simulink model "modelComposerHW"  (R2021a)
settings: Solver=VariableStepAuto  StartTime=0.0  StopTime=300  RelTol=1e-3
undefined symbols (not defined in the file or in its folder): A, N
libraries: hdlBasic x24, xbsIndex_r4 x1, JTAGRuntimeCosim_r4 x1
settings Model: Creator=kv25  LastModifiedBy=kv25

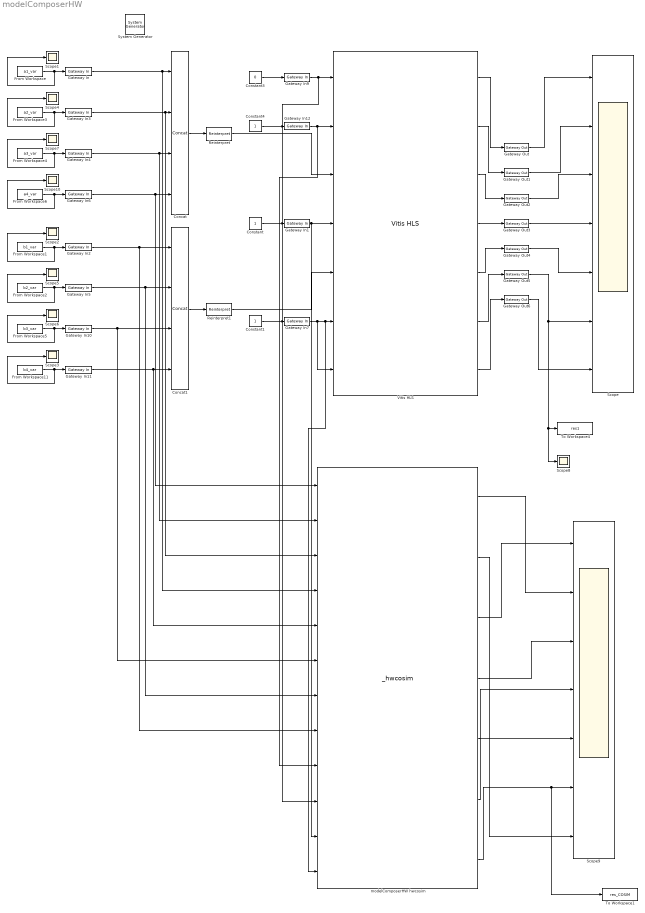
== system modelComposerHW ==
  " System Generator" : xbsIndex_r4/ System Generator  Tag=genX  xilinxfamily=zynq  part=xc7z020  speed=-1  package=clg484  synthesis_tool=Vivado  clock_wrapper=Clock Enables  directory=./netlist2  proj_type=Vivado  Synth_file=Vivado Synthesis Defaults  Impl_file=Vivado Implementation Defaults  testbench=off  simulink_period=1  sysclk_period=10  dcm_input_clock_period=10  incr_netlist=off  trim_vbits=Everywhere in SubSystem  dbl_ovrd=According to Block Masks  core_generation=According to Block Masks  run_coregen=off  deprecated_control=off  eval_field=0  block_type=sysgen
  Concat : hdlBasic/Concat  num_inputs=4  XmcBlockStatus=1  maskContainerNames=group1  block_type=concat  block_config=sysgen:Concat_config
  Concat1 : hdlBasic/Concat  num_inputs=4  XmcBlockStatus=1  maskContainerNames=group1  block_type=concat  block_config=sysgen:Concat_config
  Constant : Constant
  Constant1 : Constant
  Constant3 : Constant  Value=0
  Constant4 : Constant
  From Workspace : FromWorkspace  VariableName=a1_var
  From Workspace1 : FromWorkspace  VariableName=b1_var
  From Workspace11 : FromWorkspace  VariableName=b4_var
  From Workspace2 : FromWorkspace  VariableName=b2_var
  From Workspace3 : FromWorkspace  VariableName=a2_var
  From Workspace4 : FromWorkspace  VariableName=a3_var
  From Workspace5 : FromWorkspace  VariableName=b3_var
  From Workspace6 : FromWorkspace  VariableName=a4_var
  Gateway In{,2..6,10..11} (8 alike) : hdlBasic/Gateway In  gui_display_data_type=Fixed-point  arith_type=Unsigned  n_bits=16  bin_pt=0  preci_type=Single  exp_width=8  frac_width=24  rows=1  columns=1  quantization="Round  (unbiased: +/- Inf)"  overflow=Saturate  period=1  UseAsADC=off  ADCChannel='1'  interface=None  automatic_assignment=on  address_offset=hex2dec('00')  intf_name=''  intf_description=''  default_value=0  timing_constraint=None  locs_specified=off  LOCs={}  io_standard={}  inherit_from_input=off  hdl_port=on  XmcBlockStatus=1  maskContainerNames=group4  block_type=gatewayin  block_config=sysgen:gateway_in_config  block_width_w=590  block_height_w=620  block_width=640  block_height=850
  Gateway In{1,7,9,12} (4 alike) : hdlBasic/Gateway In  gui_display_data_type=Boolean  arith_type=Boolean  n_bits=16  bin_pt=0  preci_type=Single  exp_width=8  frac_width=24  rows=1  columns=1  quantization="Round  (unbiased: +/- Inf)"  overflow=Saturate  period=1  UseAsADC=off  ADCChannel='1'  interface=None  automatic_assignment=on  address_offset=hex2dec('00')  intf_name=''  intf_description=''  default_value=0  timing_constraint=None  locs_specified=off  LOCs={}  io_standard={}  inherit_from_input=off  hdl_port=on  XmcBlockStatus=1  maskContainerNames=group4  block_type=gatewayin  block_config=sysgen:gateway_in_config  block_width_w=590  block_height_w=620  block_width=640  block_height=850
  Gateway Out{,1..6} (7 alike) : hdlBasic/Gateway Out  inherit_from_input=off  hdl_port=on  rows=1  columns=1  UseAsDAC=off  DACChannel='1'  interface=None  automatic_assignment=on  address_offset=hex2dec('00')  intf_name=''  intf_description=''  timing_constraint=None  locs_specified=off  LOCs={}  io_standard={}  XmcBlockStatus=1  maskContainerNames=group4  block_type=gatewayout  block_config=sysgen:gateway_out_config  block_width_w=590  block_height_w=620  block_width=620  block_height=750
  Reinterpret : hdlBasic/Reinterpret  force_arith_type=on  arith_type=Unsigned  force_bin_pt=off  bin_pt=0  XmcBlockStatus=1  maskContainerNames=group1  block_type=reinterpret  block_config=sysgen:Reinterpret_config
  Reinterpret1 : hdlBasic/Reinterpret  force_arith_type=on  arith_type=Unsigned  force_bin_pt=off  bin_pt=0  XmcBlockStatus=1  maskContainerNames=group1  block_type=reinterpret  block_config=sysgen:Reinterpret_config
  Scope : Scope  NumInputPorts=7
  Scope{1..8,10} (9 alike) : Scope
  Scope9 : Scope  NumInputPorts=7
  To Workspace1 : ToWorkspace  VariableName=res_COSIM  SaveFormat=Timeseries  SampleTime=-1
  To Workspace4 : ToWorkspace  VariableName=res1  SaveFormat=Timeseries  SampleTime=-1
  Vitis HLS : hdlBasic/Vitis HLS  anytable='.\Vitis_HLS\matrixmul\solution1'  fast_sim=on  display_datatype=off  rate_propagation_method=Simulink system period  model_file_path=''  latency=1  block_type=vitis_hls
      settings: infoedit=This block allows including C,C++ and SystemC source files in System Generator for DSP designs.
  modelComposerHW hwcosim : JTAGRuntimeCosim_r4/_hwcosim  clkSrc=Single Stepped  hasCombinationalPath=on  bitfileName=C:\ELEC522\venaik\Project3\project3\netlist2\modelcomposerhw.bit  skipConfig=off  dispPartInfo=off  useZynqReconfigScript=on  cable=Auto Detect  speed=N/A  cablePort=N/A  cableLocation=Local  shareCable=off  xmp=[]  software_settings=[]  design_xtable=|  binDir=[]  engineDll=JTAGCosimEngine.dll  cableWaitTime=10  bscanPos=-1  IRLengths=[]  useWaitBox=1  hasBufgmux=on  Scheme=Cosim  useCmdProc=1  hasProc=0  useImpact=0  printLogFile=0  userChain=2  XmcBlockStatus=0  maskContainerNames=tabcontainer1  block_type=jtagcosim  block_config=Sysgen:hwcosim_block_config
      | {
      |     'clkWrapper' => 'modelcomposerhw',
      |     'burstMode' => false,
      |     'burstFifoDepth' => '1024',
      |     'shared_memories' => {},
      |     'clocksGcd' => 1,
      |     'device' => {
      |       'family' => 'zynq',
      |       'part' => 'xc7z020',
      |       'package' => 'clg484',
      |       'speed' => '-1',
      |     },
      |     'ports' => {
      |       'gateway_in6' => {
      |         'direction' => 'in',
      |         'width' => 16,
      |         'name' => 'gateway_in6',
      |         'period' => 1,
      |         'icon_text' => 'Gateway In6',
      |         'type' => 'UFix_16_0',
      |         'arithmetic_type' => 'xlUnsigned',
      |         'dat_file' => 'modelcomposerhw_gateway_in6.dat',
      |         'bin_pt' => 0,
      |         'addr_offset' => 0,
      |         'bd_port_index' => 0,
      |       },
      |       'gateway_in4' => {
      |         'direction' => 'in',
      |         'width' => 16,
      |         'name' => 'gateway_in4',
      |         'period' => 1,
      |         'icon_text' => 'Gateway In4',
      |         'type' => 'UFix_16_0',
      |         'arithmetic_type' => 'xlUnsigned',
      |         'dat_file' => 'modelcomposerhw_gateway_in4.dat',
      |         'bin_pt' => 0,
      |         'addr_offset' => 4,
      |         'bd_port_index' => 1,
      |       },
      |       'gateway_in3' => {
      |         'direction' => 'in',
      |         'width' => 16,
      |         'name' => 'gateway_in3',
      |         'period' => 1,
      |         'icon_text' => 'Gateway In3',
      |         'type' => 'UFix_16_0',
      |         'arithmetic_type' => 'xlUnsigned',
      |         'dat_file' => 'modelcomposerhw_gateway_in3.dat',
      |         'bin_pt' => 0,
      |         'addr_offset' => 8,
      |         'bd_port_index' => 2,
      |       },
      |       'gateway_in' => {
      |         'direction' => 'in',
      |         'width' => 16,
      |         'name' => 'gateway_in',
      |         'period' => 1,
      |         'icon_text' => 'Gateway In',
      |         'type' => 'UFix_16_0',
      |         'arithmetic_type' => 'xlUnsigned',
      |         'dat_file' => 'modelcomposerhw_gateway_in.dat',
      |         'bin_pt' => 0,
      |         'addr_offset' => 12,
      |         'bd_port_index' => 3,
      |       },
      |       'gateway_in11' => {
      |         'direction' => 'in',
      |         'width' => 16,
      |         'name' => 'gateway_in11',
      |         'period' => 1,
      |         'icon_text' => 'Gateway In11',
      |         'type' => 'UFix_16_0',
      |         'arithmetic_type' => 'xlUnsigned',
      |         'dat_file' => 'modelcomposerhw_gateway_in11.dat',
      |         'bin_pt' => 0,
      |         'addr_offset' => 16,
      |         'bd_port_index' => 4,
      |       },
      |       'gateway_in10' => {
      |         'direction' => 'in',
      |         'width' => 16,
      |         'name' => 'gateway_in10',
      |         'period' => 1,
      |         'icon_text' => 'Gateway In10',
      |         'type' => 'UFix_16_0',
      |         'arithmetic_type' => 'xlUnsigned',
      |         'dat_file' => 'modelcomposerhw_gateway_in10.dat',
      |         'bin_pt' => 0,
      |         'addr_offset' => 20,
      |         'bd_port_index' => 5,
      |       },
      |       'gateway_in5' => {
      |         'direction' => 'in',
      |         'width' => 16,
      |         'name' => 'gateway_in5',
      |         'period' => 1,
      |         'icon_text' => 'Gateway In5',
      |         'type' => 'UFix_16_0',
      |         'arithmetic_type' => 'xlUnsigned',
      |         'dat_file' => 'modelcomposerhw_gateway_in5.dat',
      |         'bin_pt' => 0,
      |         'addr_offset' => 24,
      |         'bd_port_index' => 6,
      |       },
      |       'gateway_in2' => {
      |         'direction' => 'in',
      |         'width' => 16,
      |         'name' => 'gateway_in2',
      |         'period' => 1,
      |         'icon_text' => 'Gateway In2',
      |         'type' => 'UFix_16_0',
      |         'arithmetic_type' => 'xlUnsigned',
      |         'dat_file' => 'modelcomposerhw_gateway_in2.dat',
      |         'bin_pt' => 0,
      |         'addr_offset' => 28,
      |         'bd_port_index' => 7,
      |       },
      |       'gateway_in12' => {
      |         'direction' => 'in',
      |         'width' => 1,
      |         'name' => 'gateway_in12',
      |         'period' => 1,
      |         'icon_text' => 'Gateway In12',
      |         'type' => 'Bool',
      |         'arithmetic_type' => 'xlUnsigned',
      |         'dat_file' => 'modelcomposerhw_gateway_in12.dat',
      |         'bin_pt' => 0,
      |         'addr_offset' => 32,
      |         'bd_port_index' => 8,
      |       },
      |       'gateway_in9' => {
      |         'direction' => 'in',
      |         'width' => 1,
      |         'name' => 'gateway_in9',
      |         'period' => 1,
      |         'icon_text' => 'Gateway In9',
      |         'type' => 'Bool',
      |         'arithmetic_type' => 'xlUnsigned',
      |         'dat_file' => 'modelcomposerhw_gateway_in9.dat',
      |         'bin_pt' => 0,
      |         'addr_offset' => 36,
      |         'bd_port_index' => 9,
      |       },
      |       'gateway_in1' => {
      |         'direction' => 'in',
      |         'width' => 1,
      |         'name' => 'gateway_in1',
      |         'period' => 1,
      |         'icon_text' => 'Gateway In1',
      |         'type' => 'Bool',
      |         'arithmetic_type' => 'xlUnsigned',
      |         'dat_file' => 'modelcomposerhw_gateway_in1.dat',
      |         'bin_pt' => 0,
      |         'addr_offset' => 40,
      |         'bd_port_index' => 10,
      |       },
      |       'gateway_in7' => {
      |         'direction' => 'in',
      |         'width' => 1,
      |         'name' => 'gateway_in7',
      |         'period' => 1,
      |         'icon_text' => 'Gateway In7',
      |         'type' => 'Bool',
      |         'arithmetic_type' => 'xlUnsigned',
      |         'dat_file' => 'modelcomposerhw_gateway_in7.dat',
      |         'bin_pt' => 0,
      |         'addr_offset' => 44,
      |         'bd_port_index' => 11,
      |       },
      |       'gateway_out1' => {
      |         'direction' => 'out',
      |         'width' => 1,
      |         'name' => 'gateway_out1',
      |         'period' => 1,
      |         'icon_text' => 'Gateway Out1',
      |         'type' => 'Bool',
      |         'arithmetic_type' => 'xlUnsigned',
      |         'dat_file' => 'modelcomposerhw_gateway_out1.dat',
      |         'bin_pt' => 0,
      |         'addr_offset' => 48,
      |         'bd_port_index' => 0,
      |       },
      |       'gateway_out6' => {
      |         'direction' => 'out',
      |         'width' => 1,
      |         'name' => 'gateway_out6',
      |         'period' => 1,
      |         'icon_text' => 'Gateway Out6',
      |         'type' => 'Bool',
      |         'arithmetic_type' => 'xlUnsigned',
      |         'dat_file' => 'modelcomposerhw_gateway_out6.dat',
      |         'bin_pt' => 0,
      |         'addr_offset' => 52,
      |         'bd_port_index' => 1,
      |       },
      |       'gateway_out' => {
      |         'direction' => 'out',
      |         'width' => 1,
      |         'name' => 'gateway_out',
      |         'period' => 1,
      |         'icon_text' => 'Gateway Out',
      |         'type' => 'Bool',
      |         'arithmetic_type' => 'xlUnsigned',
      |         'dat_file' => 'modelcomposerhw_gateway_out.dat',
      |         'bin_pt' => 0,
      |         'addr_offset' => 56,
      |         'bd_port_index' => 2,
      |       },
      |       'gateway_out2' => {
      |         'direction' => 'out',
      |         'width' => 1,
      |         'name' => 'gateway_out2',
      |         'period' => 1,
      |         'icon_text' => 'Gateway Out2',
      |         'type' => 'Bool',
      |         'arithmetic_type' => 'xlUnsigned',
      |         'dat_file' => 'modelcomposerhw_gateway_out2.dat',
      |         'bin_pt' => 0,
      |         'addr_offset' => 60,
      |         'bd_port_index' => 3,
      |       },
      |       'gateway_out3' => {
      |         'direction' => 'out',
      |         'width' => 1,
      |         'name' => 'gateway_out3',
      |         'period' => 1,
      |         'icon_text' => 'Gateway Out3',
      |         'type' => 'Bool',
      |         'arithmetic_type' => 'xlUnsigned',
      |         'dat_file' => 'modelcomposerhw_gateway_out3.dat',
      |         'bin_pt' => 0,
      |         'addr_offset' => 64,
      |         'bd_port_index' => 4,
      |       },
      |       'gateway_out4' => {
      |         'direction' => 'out',
      |         'width' => 1,
      |         'name' => 'gateway_out4',
      |         'period' => 1,
      |         'icon_text' => 'Gateway Out4',
      |         'type' => 'Bool',
      |         'arithmetic_type' => 'xlUnsigned',
      |         'dat_file' => 'modelcomposerhw_gateway_out4.dat',
      |         'bin_pt' => 0,
      |         'addr_offset' => 68,
      |         'bd_port_index' => 5,
      |       },
      |       'gateway_out5' => {
      |         'direction' => 'out',
      |         'width' => 32,
      |         'name' => 'gateway_out5',
      |         'period' => 1,
      |         'icon_text' => 'Gateway Out5',
      |         'type' => 'UFix_32_0',
      |         'arithmetic_type' => 'xlUnsigned',
      |         'dat_file' => 'modelcomposerhw_gateway_out5.dat',
      |         'bin_pt' => 0,
      |         'addr_offset' => 72,
      |         'bd_port_index' => 6,
      |       },
      |     },
      |   }
  wires:
  From Workspace4/1 -> Scope7/1, Gateway In4/1
  From Workspace6/1 -> Scope10/1, Gateway In6/1
  From Workspace/1 -> Scope1/1, Gateway In/1
  From Workspace3/1 -> Scope4/1, Gateway In3/1
  Gateway In/1 -> modelComposerHW hwcosim/4, Concat/1
  Gateway In6/1 -> modelComposerHW hwcosim/1, Concat/4
  Gateway In4/1 -> modelComposerHW hwcosim/2, Concat/3
  Gateway In3/1 -> modelComposerHW hwcosim/3, Concat/2
  Gateway In10/1 -> modelComposerHW hwcosim/6, Concat1/3
  Gateway In11/1 -> modelComposerHW hwcosim/5, Concat1/4
  Gateway In2/1 -> modelComposerHW hwcosim/8, Concat1/1
  From Workspace2/1 -> Scope5/1, Gateway In5/1
  Gateway In5/1 -> modelComposerHW hwcosim/7, Concat1/2
  From Workspace11/1 -> Scope3/1, Gateway In11/1
  From Workspace5/1 -> Scope6/1, Gateway In10/1
  From Workspace1/1 -> Scope2/1, Gateway In2/1
  Concat/1 -> Reinterpret/1
  Concat1/1 -> Reinterpret1/1
  Constant/1 -> Gateway In1/1
  Gateway In1/1 -> modelComposerHW hwcosim/11, Vitis HLS/4
  Constant1/1 -> Gateway In7/1
  Gateway In7/1 -> Vitis HLS/7, modelComposerHW hwcosim/12, Vitis HLS/6
  Constant4/1 -> Gateway In12/1
  Constant3/1 -> Gateway In9/1
  Gateway In12/1 -> modelComposerHW hwcosim/9, Vitis HLS/2
  Gateway Out/1 -> Scope/1
  Gateway Out1/1 -> Scope/2
  Gateway Out2/1 -> Scope/3
  Gateway Out3/1 -> Scope/4
  Gateway Out4/1 -> Scope/5
  Gateway Out5/1 -> Scope/6, Scope8/1, To Workspace4/1
  Reinterpret/1 -> Vitis HLS/3
  Gateway Out6/1 -> Scope/7
  Vitis HLS/1 -> Gateway Out/1
  Vitis HLS/2 -> Gateway Out1/1
  Vitis HLS/3 -> Gateway Out2/1
  Vitis HLS/4 -> Gateway Out3/1
  Vitis HLS/5 -> Gateway Out4/1
  Vitis HLS/6 -> Gateway Out5/1
  Vitis HLS/7 -> Gateway Out6/1
  Reinterpret1/1 -> Vitis HLS/5
  Gateway In9/1 -> modelComposerHW hwcosim/10, Vitis HLS/1
  modelComposerHW hwcosim/1 -> Scope9/2
  modelComposerHW hwcosim/3 -> Scope9/1
  modelComposerHW hwcosim/2 -> Scope9/7
  modelComposerHW hwcosim/7 -> To Workspace1/1, Scope9/6
  modelComposerHW hwcosim/6 -> Scope9/5
  modelComposerHW hwcosim/5 -> Scope9/4
  modelComposerHW hwcosim/4 -> Scope9/3
